simulink model "Q7_2"  (R2020b)
settings: Solver=VariableStepAuto  StartTime=0.0  StopTime=10.0  RelTol=1e-3
settings Model: Creator=Javad  LastModifiedBy=Javad

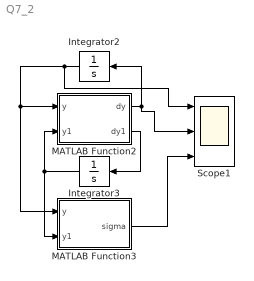
== system Q7_2 ==
  Integrator2 : Integrator  InitialCondition=1
  Integrator3 : Integrator  InitialCondition=1
  MATLAB Function2 : MATLAB Function  TreatAsAtomicUnit=on
  MATLAB Function3 : MATLAB Function  TreatAsAtomicUnit=on
  Scope1 : Scope  NumInputPorts=3
  wires:
  Integrator3/1 -> MATLAB Function3/2(y1), MATLAB Function2/2(y1)
  Integrator2/1 -> Scope1/1, MATLAB Function3/1(y), MATLAB Function2/1(y)
  MATLAB Function2/1(dy) -> Integrator2/1, Scope1/2
  MATLAB Function2/2(dy1) -> Integrator3/1
  MATLAB Function3/1(sigma) -> Scope1/3

== matlab function Q7_2/MATLAB Function3 ==
  data: y input; sigma output; y1 input
function sigma = surface1(y,y1)

sigma=y1+0.5*y;

== matlab function Q7_2/MATLAB Function2 ==
  data: y input; dy output; y1 input; dy1 output
function [dy,dy1] = fcn(y,y1)
m=1;
b=2;
k=4;
eps=10^-3;
dy=y1;
if abs(y1-0)< eps && abs(y-0)<= b/k
    dy1=-(1/m)*(-k*(y)+k*y);%=0
else
    dy1=-(1/m)*(b*sign(y1)+k*y);
end
